simulink model "matprob4"  (R2020a)
settings: Solver=VariableStepAuto  StartTime=0.0  StopTime=10.0  RelTol=1e-3
settings Model: Creator=deepa  LastModifiedBy=deepa

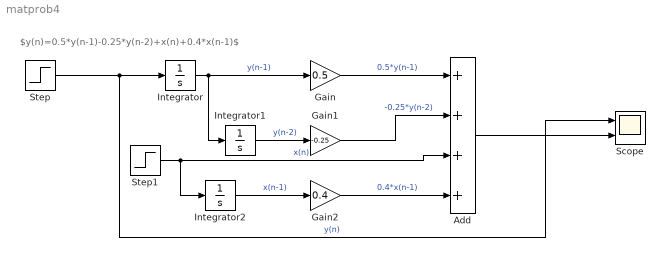
== system matprob4 ==
  note: $y(n)=0.5*y(n-1)-0.25*y(n-2)+x(n)+0.4*x(n-1)$
  Add : Sum  Inputs=++++
  Gain : Gain  Gain=0.5
  Gain1 : Gain  Gain=-0.25
  Gain2 : Gain  Gain=0.4
  Integrator : Integrator
  Integrator1 : Integrator
  Integrator2 : Integrator
  Scope : Scope  NumInputPorts=2
  Step : Step  SampleTime=0
  Step1 : Step  SampleTime=0
  wires:
  Step/1 -> Scope/1, Integrator/1  "y(n)"
  Integrator/1 -> Integrator1/1, Gain/1  "y(n-1)"
  Integrator1/1 -> Gain1/1  "y(n-2)"
  Gain/1 -> Add/1  "0.5*y(n-1)"
  Gain1/1 -> Add/2  "-0.25*y(n-2)"
  Step1/1 -> Integrator2/1, Add/3  "x(n)"
  Integrator2/1 -> Gain2/1  "x(n-1)"
  Gain2/1 -> Add/4  "0.4*x(n-1)"
  Add/1 -> Scope/2
